simulink model "MC_Phase2_Part1_Q1_Sim_v2"  (R2018b)
settings: Solver=VariableStepAuto  StartTime=0.0  StopTime=10  RelTol=1e-3
settings Model: Creator=ASUS  LastModifiedBy=1007
settings DataIOCC: ReturnWorkspaceOutputs=on

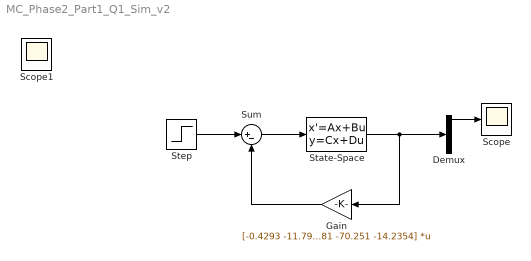
== system MC_Phase2_Part1_Q1_Sim_v2 ==
  Demux : Demux
  Gain : Gain  Gain=[-0.4293 -11.7981 -70.251 -14.2354]  Multiplication=Matrix(K*u)
  Scope : Scope
  State-Space : StateSpace  A=[0 1 0 0;0 -2.2626 -0.3963 0.0082;0 0 0 1;0 3.5649 16.0655 -0.3324]  B=[0;0.2263;0;-0.3565]  C=[1 0 0 0;0 1 0 0;0 0 1 0;0 0 0 1]  D=[0;0;0;0]  InitialCondition=0
  Step : Step  SampleTime=0
  Sum : Sum  Inputs=|+-
  Scope1 : Scope
  wires:
  State-Space/1 -> Gain/1, Demux/1
  Gain/1 -> Sum/2
  Sum/1 -> State-Space/1
  Step/1 -> Sum/1
  Demux/1 -> Scope/1
